simulink model "autoMBD_example_PI_MultirateMultitasking"  (R2020b)
settings: Solver=FixedStepAuto  StartTime=0.0  StopTime=10.0  FixedStep=0.0001  RelTol=1e-3  EnableMultiTasking=on
undefined symbols (not defined in the file): DiscIntNeverNeededParam
settings Model: Creator=k  LastModifiedBy=k
settings SolverCC: AutoInsertRateTranBlk=on
settings OptimizationCC: DefaultParameterBehavior=Inlined  EnhancedBackFolding=on  PassReuseOutputArgsAs=Individual arguments  ZeroExternalMemoryAtStartup=off  ZeroInternalMemoryAtStartup=off  OptimizeBlockOrder=speed  DifferentSizesBufferReuse=on  OptimizationCustomize=off  EfficientTunableParamExpr=on
settings DebuggingCC: ParameterTunabilityLossMsg=error
settings SFSimCC: MATLABDynamicMemAlloc=off
settings RTWCC: Description=Embedded Coder  SystemTargetFile=ert.tlc  GenCodeOnly=on  TemplateMakefile=ert_default_tmf
settings CodeAppCC: ForceParamTrailComments=on  IgnoreCustomStorageClasses=off  OperatorAnnotations=on  SimulinkDataObjDesc=on  SFDataObjDesc=on  InsertBlockDesc=on
settings ERTTargetCC: TargetLangStandard=C99 (ISO)  GenerateSampleERTMain=on  InlinedParameterPlacement=NonHierarchical  ERTCustomFileTemplate=example_file_process.tlc

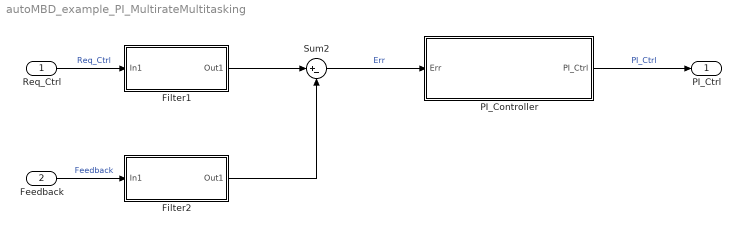
== system autoMBD_example_PI_MultirateMultitasking ==
  Req_Ctrl : Inport
  Feedback : Inport  Port=2
  Filter1 : Subsystem  TreatAsAtomicUnit=on  RTWFcnName=Filter1
      settings: RTWSystemCode=Nonreusable function  RTWFcnNameOpts=User specified
  Filter2 : Subsystem  TreatAsAtomicUnit=on  RTWFcnName=Filter2
      settings: RTWSystemCode=Nonreusable function  RTWFcnNameOpts=User specified
  PI_Controller : Subsystem  TreatAsAtomicUnit=on  SystemSampleTime=0.001  RTWFcnName=PI_Controller
      settings: RTWSystemCode=Nonreusable function  RTWFcnNameOpts=User specified
  Sum2 : Sum  Inputs=|+-
  PI_Ctrl : Outport
  wires:
  Req_Ctrl/1 -> Filter1/1(In1)  "Req_Ctrl"
  Feedback/1 -> Filter2/1(In1)  "Feedback"
  Sum2/1 -> PI_Controller/1(Err)  "Err"
  PI_Controller/1(PI_Ctrl) -> PI_Ctrl/1  "PI_Ctrl"
  Filter1/1(Out1) -> Sum2/1
  Filter2/1(Out1) -> Sum2/2

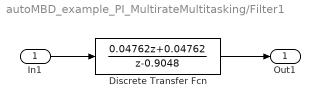
== system autoMBD_example_PI_MultirateMultitasking/Filter1 ==
  In1 : Inport
  Discrete Transfer Fcn : DiscreteTransferFcn  Numerator=[0.04762 0.04762]  Denominator=[1 -0.9048]  SampleTime=0.0001
  Out1 : Outport
  wires:
  In1/1 -> Discrete Transfer Fcn/1
  Discrete Transfer Fcn/1 -> Out1/1

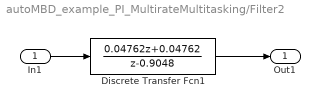
== system autoMBD_example_PI_MultirateMultitasking/Filter2 ==
  In1 : Inport
  Discrete Transfer Fcn1 : DiscreteTransferFcn  Numerator=[0.04762 0.04762]  Denominator=[1 -0.9048]  SampleTime=0.0002
  Out1 : Outport
  wires:
  In1/1 -> Discrete Transfer Fcn1/1
  Discrete Transfer Fcn1/1 -> Out1/1

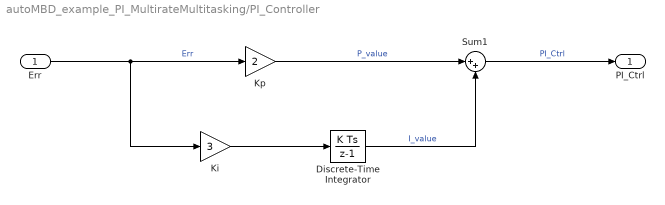
== system autoMBD_example_PI_MultirateMultitasking/PI_Controller ==
  Err : Inport  SampleTime=0.001
  Discrete-Time Integrator : DiscreteIntegrator  SampleTime=0.001  ICPrevOutput=DiscIntNeverNeededParam  ICPrevScaledInput=DiscIntNeverNeededParam
  Ki : Gain  Gain=3
  Kp : Gain  Gain=2
  Sum1 : Sum  Inputs=|++
  PI_Ctrl : Outport
  wires:
  Sum1/1 -> PI_Ctrl/1  "PI_Ctrl"
  Err/1 -> Ki/1, Kp/1  "Err"
  Discrete-Time Integrator/1 -> Sum1/2  "I_value"
  Ki/1 -> Discrete-Time Integrator/1
  Kp/1 -> Sum1/1  "P_value"
